simulink model "inverter"  (R2018a)
settings: Solver=VariableStepDiscrete  StartTime=0.0  StopTime=10.0  RelTol=1e-3
libraries: powerlib x10
settings Model: Creator=Bhaskar  LastModifiedBy=Bhaskar

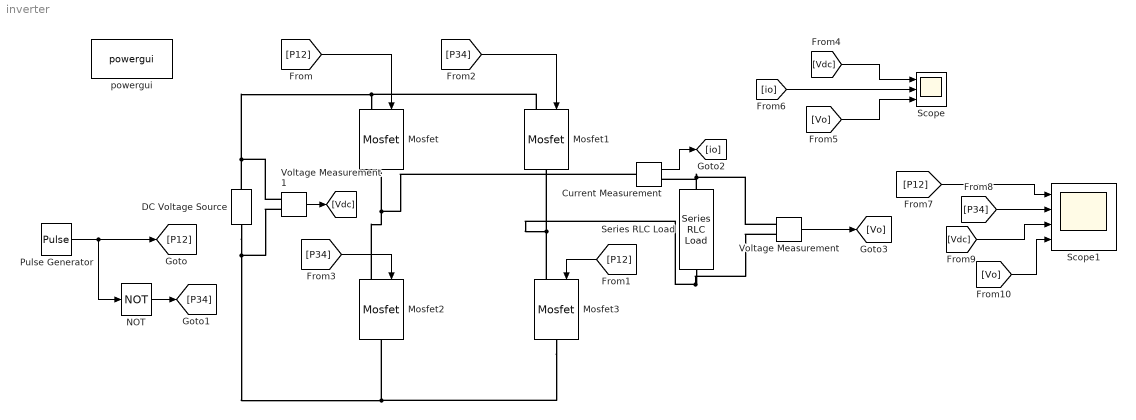
== system inverter ==
  Current Measurement : powerlib/Measurements/Current Measurement  PhasorSimulation=off  OutputType=Complex  PSBequivalent=0
  DC Voltage Source : powerlib/Electrical Sources/DC Voltage Source  Amplitude=100  Measurements=None
  Mosfet{,1..3} (4 alike) : powerlib/Power Electronics/Mosfet  Ron=0.1  Lon=0  Rd=0.01  Vfd=0  IC=0  Rs=1e5  Cs=inf  Measurements=off
  NOT : Logic  Operator=NOT  IconShape=distinctive  AllPortsSameDT=off  OutDataTypeStr=boolean
  Pulse Generator : DiscretePulseGenerator  PulseType=Time based  Period=1/50  PulseWidth=50
  Scope : Scope  NumInputPorts=3
  Scope1 : Scope  NumInputPorts=4
  Series RLC Load : powerlib/Elements/Series RLC Load  LConnTagsString=a  RConnTagsString=__new0  NominalVoltage=230  NominalFrequency=50  ActivePower=1000  InductivePower=0  CapacitivePower=0  Setx0=off  InitialVoltage=0  SetiL0=off  InitialCurrent=0  Measurements=None  LoadType=constant Z
  Voltage Measurement : powerlib/Measurements/Voltage Measurement  PhasorSimulation=off  OutputType=Complex  PSBequivalent=0
  Voltage Measurement1 : powerlib/Measurements/Voltage Measurement  PhasorSimulation=off  OutputType=Complex  PSBequivalent=0
  powergui : powerlib/powergui  Priority=1  SimulationMode=Discrete  SampleTime=50e-6  frequency=60  Iterations=50  frequencyindice=0  Pbase=100e6  ErrMax=1e-4  UnitsV=kV  UnitsW=MW  buscounter=0  FunctionMessages=off  echomessages=off  EnableUseOfTLC=off  CurrentSourceSwitches=off  DisableSnubberDevices=off  DisableRonSwitches=off  DisableVfSwitches=off  DisplayEquations=off  SolverType=Tustin/Backward Euler (TBE)  Interpol=off  ExternalGateDelay=off  methode=off  Ts=100  x0status=blocks  SPID=on  SwTol=0  HookPort=off  RestoreLinks=warning  ResistiveCurrentMeasurement=off  Frange=[0:2:500]  Ylog=off  Xlog=on  ShowGrid=off  save=off  variable=ZData  structure=0  ZoomFFT=off  StartTime=0.0  cycles=1  DisplayStyle=1  fundamental=60  FreqAxis=off  MaxFrequency=1000  frequencyindicesteady=1  RmsSteady=1  display=off
  wires:
  Pulse Generator/1 -> NOT/1, [P12]
  [P12] -> Mosfet/1
  [P12] -> Mosfet3/1
  NOT/1 -> [P34]
  [P34] -> Mosfet2/1
  [P34] -> Mosfet1/1
  Voltage Measurement1/1 -> [Vdc]
  Current Measurement/1 -> [io]
  Voltage Measurement/1 -> [Vo]
  [Vdc] -> Scope/1
  [io] -> Scope/2
  [Vo] -> Scope/3
  [P12] -> Scope1/1
  [P34] -> Scope1/2
  [Vdc] -> Scope1/3
  [Vo] -> Scope1/4
  connections:
  DC Voltage Source/RConn1 -- Voltage Measurement1/LConn1 -- Mosfet1/LConn1 -- Mosfet/LConn1
  Mosfet2/LConn1 -- Current Measurement/LConn1 -- Mosfet/RConn1
  Mosfet3/LConn1 -- Voltage Measurement/LConn2 -- Series RLC Load/LConn1 -- Mosfet1/RConn1
  DC Voltage Source/LConn1 -- Voltage Measurement1/LConn2 -- Mosfet2/RConn1 -- Mosfet3/RConn1
  Series RLC Load/RConn1 -- Voltage Measurement/LConn1 -- Current Measurement/RConn1
